simulink model "cdo_vawt_simscape_plant"  (R2025b)
settings: Solver=ode23t  StartTime=0.0  StopTime=60  RelTol=1e-3
libraries: fl_lib x6, nesl_utility x4
settings Model: Creator=User  LastModifiedBy=User

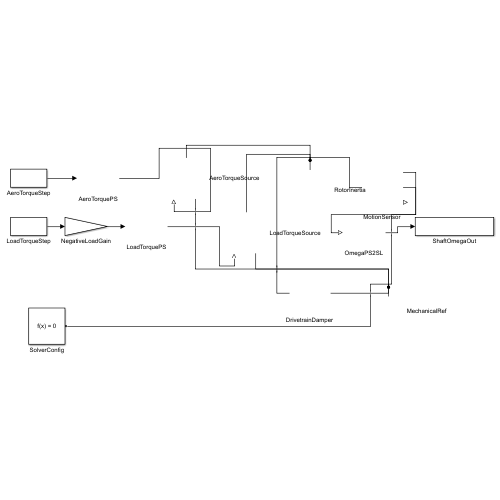
[thumbnail: Simulink's stored preview of the top-level diagram]
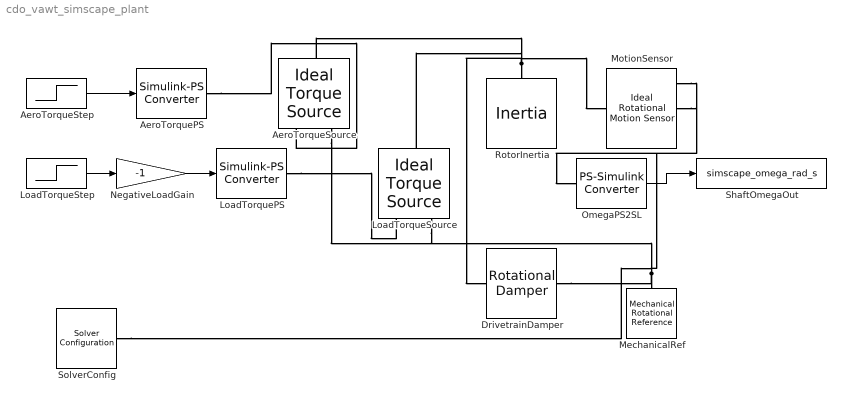
== system cdo_vawt_simscape_plant ==
  AeroTorquePS : nesl_utility/Simulink-PS Converter  PhysicalDomain=network_engine_domain  SubClassName=ps_input  LeftPortType=input  RightPortType=output  PseudoPeriodic=off  Frequencies=[]  NoiseDistribution=none  NoiseParameters=[]  Unit=N*m  AffineConversion=off  FilteringAndDerivatives=provide  SimscapeFilterOrder=1  InputFilterTimeConstant=0.001  UdotUserProvided=0
  AeroTorqueSource : fl_lib/Mechanical/Mechanical Sources/Ideal Torque Source
  AeroTorqueStep : Step  Time=5  After=6  SampleTime=0
  DrivetrainDamper : fl_lib/Mechanical/Rotational Elements/Rotational Damper  D=0.08 N*m*s/rad  w_specify=off  w_priority=None  w=0 rad/s  w_nominal_specify=off  w_nominal_value=1  w_nominal_unit=rad/s  t_specify=off  t_priority=None  t=0 N*m  t_nominal_specify=off  t_nominal_value=1  t_nominal_unit=N*m
  LoadTorquePS : nesl_utility/Simulink-PS Converter  PhysicalDomain=network_engine_domain  SubClassName=ps_input  LeftPortType=input  RightPortType=output  PseudoPeriodic=off  Frequencies=[]  NoiseDistribution=none  NoiseParameters=[]  Unit=N*m  AffineConversion=off  FilteringAndDerivatives=provide  SimscapeFilterOrder=1  InputFilterTimeConstant=0.001  UdotUserProvided=0
  LoadTorqueSource : fl_lib/Mechanical/Mechanical Sources/Ideal Torque Source
  LoadTorqueStep : Step  Time=10  After=2  SampleTime=0
  MechanicalRef : fl_lib/Mechanical/Rotational Elements/Mechanical Rotational Reference
  MotionSensor : fl_lib/Mechanical/Mechanical Sensors/Ideal Rotational Motion Sensor  reference=foundation.enum.MeasurementReference.difference  acceleration_port=false  velocity_port=true  position_port=true  wrap_angle=false  offset=0 rad
  NegativeLoadGain : Gain  Gain=-1
  OmegaPS2SL : nesl_utility/PS-Simulink Converter  PhysicalDomain=network_engine_domain  SubClassName=ps_output  LeftPortType=input  RightPortType=output  PseudoPeriodic=off  Frequencies=[]  VectorFormat=inherit  Unit=rad/s  AffineConversion=off
  RotorInertia : fl_lib/Mechanical/Rotational Elements/Inertia  inertia=12 kg*m^2  num_ports=foundation.enum.numPorts2.one  w_specify=off  w_priority=High  w=0 rad/s  w_nominal_specify=off  w_nominal_value=1  w_nominal_unit=rad/s  t_specify=off  t_priority=None  t=0 N*m  t_nominal_specify=off  t_nominal_value=1  t_nominal_unit=N*m
  ShaftOmegaOut : ToWorkspace  VariableName=simscape_omega_rad_s  SaveFormat=Structure With Time  SampleTime=-1
  SolverConfig : nesl_utility/Solver Configuration  PhysicalDomain=network_engine_domain  SubClassName=solver  LeftPortType=input  RightPortType=generic  Tones=[]  Harmonics=[]  SimulateNoise=off  Profile=off  UseLocalSampling=off  EnableSwitchedLinearOptims=on  FrequencyDomain=off  UseCCode=off  RelTol=0.001  AbsTol=0.001  MinStep=1e-09  ToWorkspace=off  RevertToSquareIcSolve=off  NumHomotopyIterations=100  PhasorMode=off  PhasorModeNumHarmonics=1  ConsistencySolver=NEWTON_XTOL_AFTER_FTOL  IndexReductionMethod=DerivativeReplacement  DoDC=off  ResidualTolerance=1e-09  ConsistencyTolSource=GLOBAL  ConsistencyAbsTol=0.001  ConsistencyRelTol=0.001  ConsistencyTolFactor=0.001  UseLocalSolver=off  LocalSolverChoice=NE_BACKWARD_EULER_ADVANCER  ResolveIndetEquations=on  FunctionEvalNumThread=1  LocalSolverSampleTime=0.001  DoFixedCost=off  MaxNonlinIter=3  MaxModeIter=2  ComputeImpulses=off  ImpulseIterations=2  LinearAlgebra=auto  LinearAlgebraNumThread=0  EquationFormulation=NE_TIME_EF  DelaysMemoryBudget=1024  AutomaticFiltering=on  FilteringTimeConstant=0.001  PartitionStorageMethod=AS_NEEDED  PartitionMemoryBudget=1024  PartitionMethod=ROBUST  MultibodyUseLocalSolver=off  MultibodyLocalSolverChoice=ODE1  MultibodyLocalSolverSampleTime=0.001
  wires:
  AeroTorqueStep/1 -> AeroTorquePS/1
  LoadTorqueStep/1 -> NegativeLoadGain/1
  NegativeLoadGain/1 -> LoadTorquePS/1
  OmegaPS2SL/1 -> ShaftOmegaOut/1
  connections:
  AeroTorquePS/RConn1 -- AeroTorqueSource/RConn1
  LoadTorquePS/RConn1 -- LoadTorqueSource/RConn1
  AeroTorqueSource/LConn1 -- LoadTorqueSource/LConn1 -- MotionSensor/LConn1 -- RotorInertia/LConn1 -- DrivetrainDamper/LConn1
  AeroTorqueSource/RConn2 -- LoadTorqueSource/RConn2 -- DrivetrainDamper/RConn1 -- MotionSensor/RConn1 -- MechanicalRef/LConn1 -- SolverConfig/RConn1
  MotionSensor/RConn2 -- OmegaPS2SL/LConn1
